simulink model "ASM_FOC_Implementation_Drive2"  (R2021a)
settings: Solver=ode3  StartTime=0.0  StopTime=t_end  FixedStep=dt  RelTol=1e-3  EnableMultiTasking=on
values from neighbouring files (symbols this model uses):
  dt = 5e-6    (= 5e-06)    [Experiment_4_Parameter.m]
  dt_omega = 5e-4    (= 0.0005)    [Experiment_4_Parameter.m]
  EncoderLines = 4096    [Experiment_4_Parameter.m]
  I_N = 4.5*sqrt(2)    [Experiment_4_Parameter.m]
  K_i_i = V_C_i/T_n_i    (= 35.4720958972)    [Experiment_4_Parameter.m]
  K_i_omega = V_C_omega/T_n_omecga_m    (= 32.203207405)    [Experiment_4_Parameter.m]
  K_i_psi = V_C_psi/T_n_psi    (= 3067.48466258)    [Experiment_4_Parameter.m]
  K_p_i = V_C_i    (= 0.195882352941)    [Experiment_4_Parameter.m]
  K_p_omega = V_C_omega    (= 0.32203207405)    [Experiment_4_Parameter.m]
  K_p_psi = V_C_psi    (= 359.636132854)    [Experiment_4_Parameter.m]
  L_m = 0.326    [Experiment_4_Parameter.m]
  L_r = 0.340    (= 0.34)    [Experiment_4_Parameter.m]
  L_s = 0.340    (= 0.34)    [Experiment_4_Parameter.m]
  L_sigma_r = L_r - L_m    (= 0.014)    [Experiment_4_Parameter.m]
  L_sigma_s = L_s - L_m    (= 0.014)    [Experiment_4_Parameter.m]
  M_MN = P_N / omega_N    (= 7.26936072254)    [Experiment_4_Parameter.m]
  n_Igain = 0.075    [Experiment_4_Parameter.m]
  n_Imax = 0.15    [Experiment_4_Parameter.m]
  n_Imin = -n_Imax    (= -0.15)    [Experiment_4_Parameter.m]
  N_N = 2890    [Experiment_4_Parameter.m]
  p = 1    [Experiment_4_Parameter.m]
  Psi_rN = 0.95    [Experiment_4_Parameter.m]
  R_r = 2.9    [Experiment_4_Parameter.m]
  R_s = 2.3    [Experiment_4_Parameter.m]
  sigma = (L_s*L_r - L_m^2)/(L_s*L_r)    (= 0.0806574394464)    [Experiment_4_Parameter.m]
  T_c = 1/4000    (= 0.00025)    [Experiment_4_Parameter.m]
  Theta_M = 0.0022    [Experiment_4_Parameter.m]
  U_dc = 560    [Experiment_4_Parameter.m]
libraries: spsIGBTDiodeLib x6, simulink x3, spsDCVoltageSourceLib x2, spsVoltageMeasurementLib x2, spsGroundLib x1, spspowerguiLib x1, eeTransforms x1
settings Model: Creator=julien  LastModifiedBy=go25bes
settings SolverCC: AlgebraicLoopSolver=TrustRegion
settings DataIOCC: LimitDataPoints=on  SaveFormat=Array  ReturnWorkspaceOutputs=off
settings OptimizationCC: ExpressionDepthLimit=2147483647  LifeSpan=inf
settings DebuggingCC: UnderspecifiedInitializationDetection=Classic  MergeDetectMultiDrivingBlocksExec=none  SolverPrmCheckMsg=warning  MultiTaskRateTransMsg=warning  StateNameClashWarn=warning  SFUnexpectedBacktrackingDiag=warning  SFNoUnconditionalDefaultTransitionDiag=warning  SFExecutionAtInitializationDiag=none  SFMachineParentedDataDiag=warning  ArithmeticOperatorsInVariantConditions=warning
settings HardwareCC: ProdBitPerPointer=32  ProdBitPerSizeT=32  ProdBitPerPtrDiffT=32  ProdLargestAtomicFloat=None  ProdIntDivRoundTo=Undefined  ProdEndianess=Unspecified  ProdWordSize=32  ProdHWDeviceType=32-bit Generic
settings ModelReferenceCC: PropagateSignalLabelsOutOfModel=off
settings SFSimCC: SimUseLocalCustomCode=off  CustomCodeUndefinedFunction=UseInterfaceOnly
settings RTWCC: RTWUseLocalCustomCode=off
settings CodeAppCC: StateflowObjectComments=on
settings GRTTargetCC: TargetLangStandard=C89/C90 (ANSI)
settings ConfigComp: CovMetricSettings=dw  CovSaveCumulativeToWorkspaceVar=on  CovSaveSingleToWorkspaceVar=on  CovExternalEMLEnable=off  CovSFcnEnable=off
settings SimscapeCC: SimscapeNormalizeSystem=off

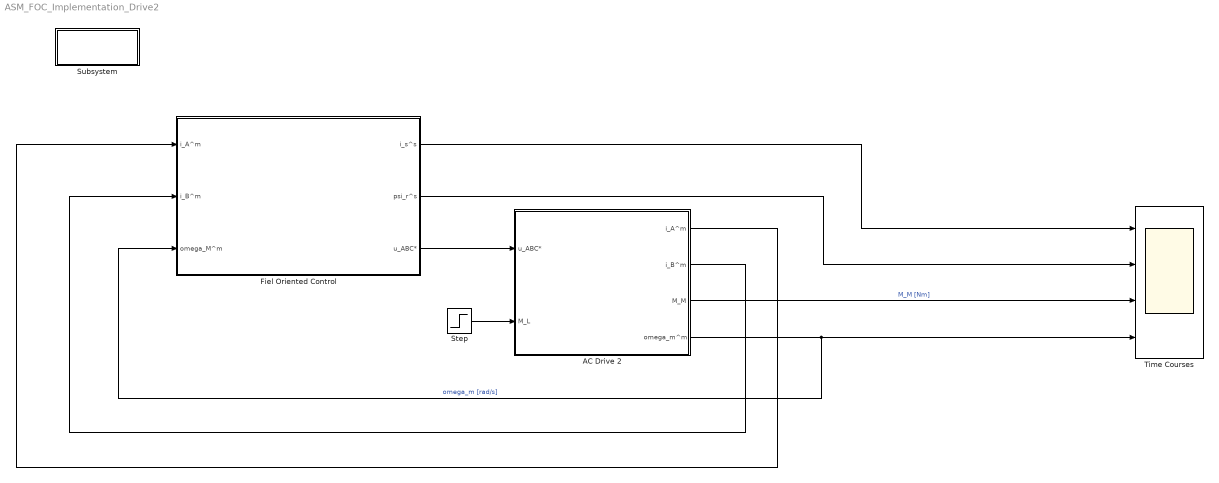
== system ASM_FOC_Implementation_Drive2 ==
  AC Drive 2 : Subsystem
  Fiel Oriented Control : Subsystem
  Step : Step  Time=0.5  After=0.5*M_MN  SampleTime=0
  Subsystem : Subsystem
      settings: OpenFcn=Experiment_4_Parameter
      mask Display: disp('Initialize\n (doppelklicken)')
  Time Courses : Scope  NumInputPorts=4
  wires:
  AC Drive 2/4(omega_m^m) -> Time Courses/4, Fiel Oriented Control/3(omega_M^m)  "omega_m [rad/s]"
  AC Drive 2/3(M_M) -> Time Courses/3  "M_M [Nm]"
  AC Drive 2/1(i_A^m) -> Fiel Oriented Control/1(i_A^m)
  AC Drive 2/2(i_B^m) -> Fiel Oriented Control/2(i_B^m)
  Fiel Oriented Control/1(i_s^s) -> Time Courses/1
  Fiel Oriented Control/3(u_ABC*) -> AC Drive 2/1(u_ABC*)
  Fiel Oriented Control/2(psi_r^s) -> Time Courses/2
  Step/1 -> AC Drive 2/2(M_L)

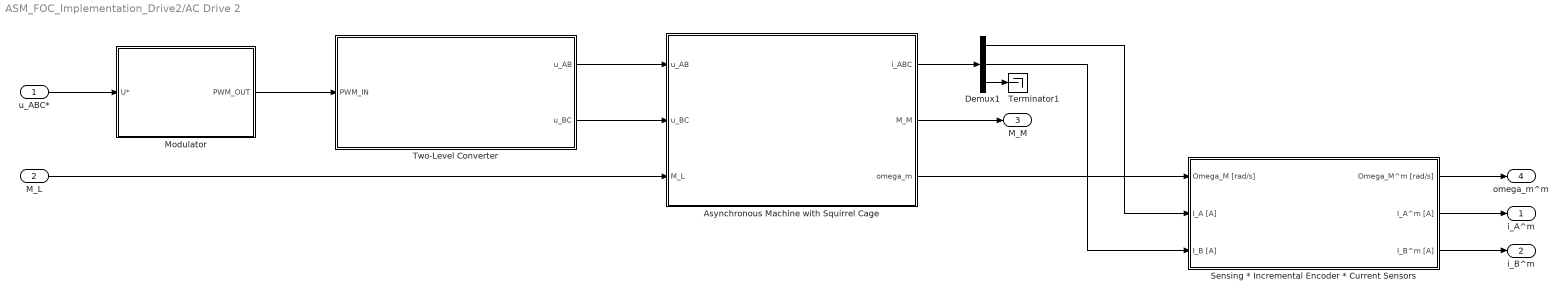
== system ASM_FOC_Implementation_Drive2/AC Drive 2 ==
  u_ABC* : Inport
  M_L : Inport  Port=2
  Asynchronous Machine with Squirrel Cage : Subsystem
  Demux1 : Demux  Outputs=3
  Modulator : Subsystem
  Sensing * Incremental Encoder * Current Sensors : Subsystem
  Terminator1 : Terminator
  Two-Level Converter : Subsystem
  i_A^m : Outport
  i_B^m : Outport  Port=2
  M_M : Outport  Port=3
  omega_m^m : Outport  Port=4
  wires:
  Asynchronous Machine with Squirrel Cage/2(M_M) -> M_M/1
  M_L/1 -> Asynchronous Machine with Squirrel Cage/3(M_L)
  u_ABC*/1 -> Modulator/1(U*)
  Modulator/1(PWM_OUT) -> Two-Level Converter/1(PWM_IN)
  Two-Level Converter/1("u_AB ") -> Asynchronous Machine with Squirrel Cage/1(u_AB)
  Two-Level Converter/2("u_BC ") -> Asynchronous Machine with Squirrel Cage/2(u_BC)
  Asynchronous Machine with Squirrel Cage/1(i_ABC) -> Demux1/1
  Demux1/3 -> Terminator1/1
  Sensing * Incremental Encoder * Current Sensors/1(Omega_M^m [rad/s]) -> omega_m^m/1
  Sensing * Incremental Encoder * Current Sensors/2(I_A^m [A]) -> i_A^m/1
  Demux1/2 -> Sensing * Incremental Encoder * Current Sensors/3(I_B [A])
  Demux1/1 -> Sensing * Incremental Encoder * Current Sensors/2(I_A [A])
  Asynchronous Machine with Squirrel Cage/3(omega_m) -> Sensing * Incremental Encoder * Current Sensors/1(Omega_M [rad/s])
  Sensing * Incremental Encoder * Current Sensors/3(I_B^m [A]) -> i_B^m/1

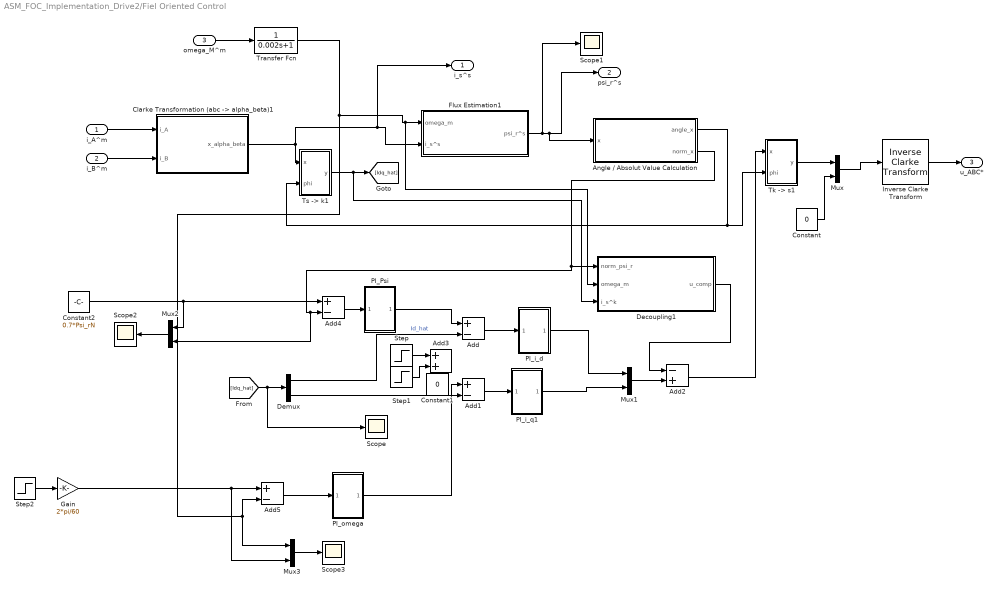
== system ASM_FOC_Implementation_Drive2/Fiel Oriented Control ==
  i_A^m : Inport
  i_B^m : Inport  Port=2
  omega_M^m : Inport  Port=3
  Add{,1,4..5} (4 alike) : Sum  Inputs=+-
  Add2 : Sum  Inputs=-+
  Add3 : Sum
  "Angle / Absolut Value Calculation " : Subsystem
  "Clarke Transformation (abc -> alpha_beta)1" : Subsystem
  Constant : Constant  Value=0
  Constant1 : Constant  Value=0
  Constant2 : Constant  Value=0.7*Psi_rN
  Decoupling1 : Subsystem
  Demux : Demux  Outputs=2
  Flux Estimation1 : Subsystem
  Gain : Gain  Gain=2*pi/60
  Inverse Clarke Transform : eeTransforms/Inverse Clarke Transform  PowerInvariant=off
      settings: SourceProductBaseCode=PS
  Mux{,1..3} (4 alike) : Mux  Inputs=2
  PI_Psi : Subsystem
  PI_i_d : Subsystem
  PI_i_q1 : Subsystem
  PI_omega : Subsystem
  Scope{,1..3} (4 alike) : Scope
  Step : Step  Time=0.6  After=2  SampleTime=0
  Step1 : Step  Time=0.8  After=-2  SampleTime=0
  Step2 : Step  Time=0.2  After=1.1*N_N  SampleTime=0
  "Tk -> s1" : Subsystem
  Transfer Fcn : TransferFcn  Denominator=[0.002 1]
  "Ts -> k1" : Subsystem
  i_s^s : Outport
  psi_r^s : Outport  Port=2
  u_ABC* : Outport  Port=3
  wires:
  i_A^m/1 -> "Clarke Transformation (abc -> alpha_beta)1"/1(i_A)
  i_B^m/1 -> "Clarke Transformation (abc -> alpha_beta)1"/2(i_B)
  "Clarke Transformation (abc -> alpha_beta)1"/1(x_alpha_beta) -> i_s^s/1, Flux Estimation1/2(i_s^s), "Ts -> k1"/1(x)
  Flux Estimation1/1(psi_r^s) -> Scope1/1, "Angle / Absolut Value Calculation "/1(x), psi_r^s/1
  "Tk -> s1"/1(y) -> Mux/1
  "Angle / Absolut Value Calculation "/1(angle_x) -> "Ts -> k1"/2(phi), "Tk -> s1"/2(phi)
  Inverse Clarke Transform/1 -> u_ABC*/1
  Constant/1 -> Mux/2
  Mux/1 -> Inverse Clarke Transform/1
  "Ts -> k1"/1(y) -> Decoupling1/3(i_s^k), [Idq_hat]
  [Idq_hat] -> Scope/1, Demux/1
  Demux/1 -> Add/2  "Id_hat"
  Demux/2 -> Add1/2
  Add/1 -> PI_i_d/1(In1)
  PI_i_d/1(Out1) -> Mux1/1
  Add1/1 -> PI_i_q1/1(In1)
  PI_i_q1/1(Out1) -> Mux1/2
  Mux1/1 -> Add2/2
  Add2/1 -> "Tk -> s1"/1(x)
  "Angle / Absolut Value Calculation "/2(norm_x) -> Mux2/2, Add4/2, Decoupling1/1(norm_psi_r)
  Step/1 -> Add3/1
  Step1/1 -> Add3/2
  Decoupling1/1(u_comp) -> Add2/1
  Add4/1 -> PI_Psi/1(In1)
  Constant2/1 -> Mux2/1, Add4/1
  PI_Psi/1(Out1) -> Add/1
  Mux2/1 -> Scope2/1
  omega_M^m/1 -> Transfer Fcn/1
  Add5/1 -> PI_omega/1(In1)
  PI_omega/1(Out1) -> Add1/1
  Mux3/1 -> Scope3/1
  Step2/1 -> Gain/1
  Gain/1 -> Mux3/2, Add5/1
  Transfer Fcn/1 -> Mux3/1, Add5/2, Decoupling1/2(omega_m), Flux Estimation1/1(omega_m)

== system ASM_FOC_Implementation_Drive2/Subsystem ==

== system ASM_FOC_Implementation_Drive2/AC Drive 2/Asynchronous Machine with Squirrel Cage ==
  u_AB : Inport
  u_BC : Inport  Port=2
  M_L : Inport  Port=3
  Calculation of the Voltage Space Vector : Subsystem
  General AC Machine : Subsystem
  "Inverse Clarke Transformation (alpha_beta -> abc)" : Subsystem
  Rotor Voltage : Constant  Value=0
  Time Courses : Scope  NumInputPorts=5
  i_ABC : Outport
  M_M : Outport  Port=2
  omega_m : Outport  Port=3
  wires:
  Rotor Voltage/1 -> General AC Machine/2(u_r^r)
  Calculation of the Voltage Space Vector/1(u_alpha_beta) -> General AC Machine/1(u_s^s)
  General AC Machine/1(i_s^s) -> Time Courses/1, "Inverse Clarke Transformation (alpha_beta -> abc)"/1(x_alpha_beta)  "i_s^s [A]"
  M_L/1 -> General AC Machine/3(M_L)
  General AC Machine/5(M_M) -> Time Courses/5, M_M/1  "M_M [Nm]"
  "Inverse Clarke Transformation (alpha_beta -> abc)"/1(x_ABC) -> i_ABC/1
  General AC Machine/6(omega_m) -> omega_m/1
  u_AB/1 -> Calculation of the Voltage Space Vector/1(u_AB)
  u_BC/1 -> Calculation of the Voltage Space Vector/2(u_BC)
  General AC Machine/2(psi_s^s) -> Time Courses/2  "psi_s^s [Vs]"
  General AC Machine/3(i_r^r) -> Time Courses/3  "i_r^r [A]"
  General AC Machine/4(psi_r^r) -> Time Courses/4  "psi_r^r [Vs]"

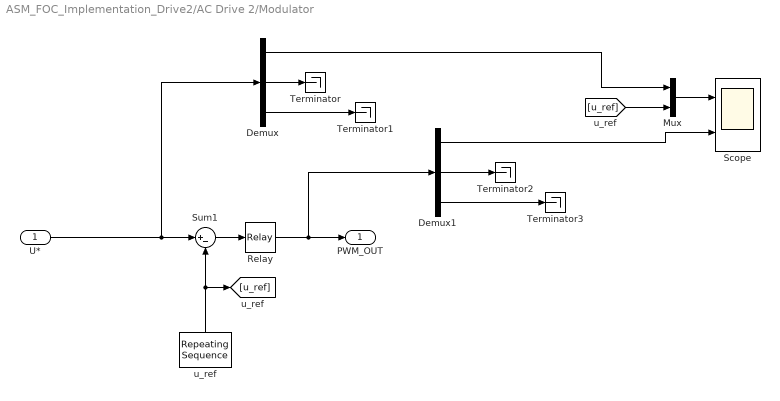
== system ASM_FOC_Implementation_Drive2/AC Drive 2/Modulator ==
  U* : Inport
  Demux : Demux  Outputs=3
  Demux1 : Demux  Outputs=3
  Mux : Mux  Inputs=2
  Relay : Relay  OnSwitchValue=1e-4  OffSwitchValue=-1e-4
  Scope : Scope  NumInputPorts=2
  Sum1 : Sum  Inputs=|+-
  Terminator{,1..3} (4 alike) : Terminator
  u_ref : simulink/Sources/Repeating Sequence  rep_seq_t="[0 T_c/2  T_c]"  rep_seq_y=[1 -1 1]
  PWM_OUT : Outport
  wires:
  Sum1/1 -> Relay/1
  Relay/1 -> Demux1/1, PWM_OUT/1
  Demux/1 -> Mux/1
  Mux/1 -> Scope/1
  u_ref/1 -> [u_ref], Sum1/2
  U*/1 -> Demux/1, Sum1/1
  Demux/2 -> Terminator/1
  Demux/3 -> Terminator1/1
  [u_ref] -> Mux/2
  Demux1/2 -> Terminator2/1
  Demux1/3 -> Terminator3/1
  Demux1/1 -> Scope/2

== system ASM_FOC_Implementation_Drive2/AC Drive 2/Sensing * Incremental Encoder * Current Sensors ==
  Omega_M [rad/s] : Inport
  I_A [A] : Inport  Port=2
  I_B [A] : Inport  Port=3
  Current Sensor : Subsystem  mask(Noise Generator){Noise_Power=0.1*dt, h_Noise=dt, V_Noise=n_Igain, Max_Noise=n_Imax*I_N, Min_Noise=n_Imin*I_N}
      mask prompts: Noise_Power "Noise Power (default: 0.1*h)"; h_Noise "Noise Sampling Time (default: h)"; V_Noise "Noise Gain (Amplification)"; Max_Noise "Maximal Noise Amplitude (Saturation)"; Min_Noise "Minimal Noise Amplitude (Saturation)"
      mask help:
      | This block generates sensor noise (band limited white noise) at a noise sampling time h_Noise [s, default: h] and with a noise power Noise_Power [1, default: 0.1*h], to produce normally distributed bandlimited white noise with a maximal amplitude around 1.
      | The noise amplitude can be amplified with a noise gain V_Noise [1] and saturated with the maximal and minimal noise amplitude selection.
      | With the flag "ENABLE_NOISE" (constant) the noise output can be activated or set to zero.
      mask Display:
      | fprintf('Noise Power: %1.3f [1]\n Noise Sampling Time: %1.3f [s] \n Noise Gain: %g [1] \n Saturation: [%g,%g]'...
      |    ,Noise_Power, h_Noise, V_Noise, Min_Noise, Max_Noise);
      | port_label('input',1,'I [A]');
      | port_label('output',1,'I^m [A]');
  "Current Sensor " : Subsystem  mask(Noise Generator){Noise_Power=0.1*dt, h_Noise=dt, V_Noise=n_Igain, Max_Noise=n_Imax*I_N, Min_Noise=n_Imin*I_N}
      mask prompts: Noise_Power "Noise Power (default: 0.1*h)"; h_Noise "Noise Sampling Time (default: h)"; V_Noise "Noise Gain (Amplification)"; Max_Noise "Maximal Noise Amplitude (Saturation)"; Min_Noise "Minimal Noise Amplitude (Saturation)"
      mask help:
      | This block generates sensor noise (band limited white noise) at a noise sampling time h_Noise [s, default: h] and with a noise power Noise_Power [1, default: 0.1*h], to produce normally distributed bandlimited white noise with a maximal amplitude around 1.
      | The noise amplitude can be amplified with a noise gain V_Noise [1] and saturated with the maximal and minimal noise amplitude selection.
      | With the flag "ENABLE_NOISE" (constant) the noise output can be activated or set to zero.
      mask Display:
      | fprintf('Noise Power: %1.3f [1]\n Noise Sampling Time: %1.3f [s] \n Noise Gain: %g [1] \n Saturation: [%g,%g]'...
      |    ,Noise_Power, h_Noise, V_Noise, Min_Noise, Max_Noise);
      | port_label('input',1,'I [A]');
      | port_label('output',1,'I^m [A]');
  Inkremental-Encoder : Subsystem  mask(Noise Generator){enc_lines=EncoderLines}
      mask prompts: enc_lines "Encoder Lines"
      mask help:
      | This block generates sensor noise (band limited white noise) at a noise sampling time h_Noise [s, default: h] and with a noise power Noise_Power [1, default: 0.1*h], to produce normally distributed bandlimited white noise with a maximal amplitude around 1.
      | The noise amplitude can be amplified with a noise gain V_Noise [1] and saturated with the maximal and minimal noise amplitude selection.
      | With the flag "ENABLE_NOISE" (constant) the noise output can be activated or set to zero.
      mask Display:
      | fprintf('Encoder Lines %g [1]',enc_lines);
      | port_label('input',1,'Omega [rad/s]');
      | port_label('output',1,'Omega^m [rad/s]');
  Omega_M^m [rad/s] : Outport  InitialOutput=0
  I_A^m [A] : Outport  Port=2  InitialOutput=0
  I_B^m [A] : Outport  Port=3  InitialOutput=0
  wires:
  Omega_M [rad/s]/1 -> Inkremental-Encoder/1(Omega [rad/s])
  I_A [A]/1 -> Current Sensor/1(Input)
  I_B [A]/1 -> "Current Sensor "/1(Input)
  "Current Sensor "/1(Output (disturbed by measurement noise)) -> I_B^m [A]/1
  Current Sensor/1(Output (disturbed by measurement noise)) -> I_A^m [A]/1
  Inkremental-Encoder/1(Omega [rad/s] (disturbed by measurement noise)) -> Omega_M^m [rad/s]/1

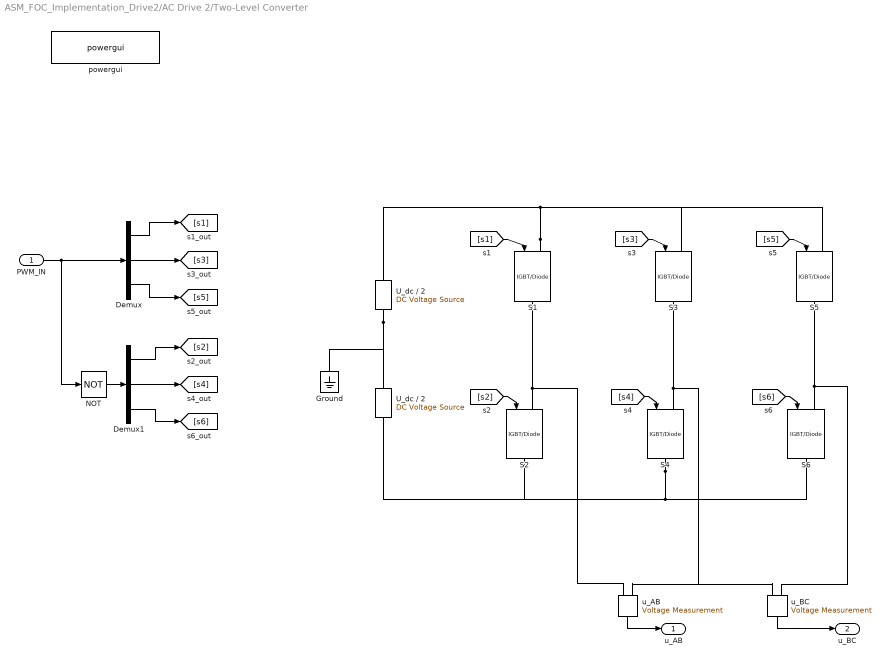
== system ASM_FOC_Implementation_Drive2/AC Drive 2/Two-Level Converter ==
  PWM_IN : Inport
  Demux : Demux  Outputs=3
  Demux1 : Demux  Outputs=3
  Ground : spsGroundLib/Ground  LConnTagsString=a
  NOT : Logic  Operator=NOT  AllPortsSameDT=off  OutDataTypeStr=boolean
  S{1..6} (6 alike) : spsIGBTDiodeLib/IGBT//Diode  Ron=1e-3  Rs=1e5  Cs=inf  Measurements=off
  U_dc / 2 : spsDCVoltageSourceLib/DC Voltage Source  Amplitude=U_dc/2  Measurements=None
  "U_dc / 2 " : spsDCVoltageSourceLib/DC Voltage Source  Amplitude=U_dc/2  Measurements=None
  powergui : spspowerguiLib/powergui  Priority=1  SimulationMode=Discrete  SampleTime=dt  frequency=60  Iterations=50  frequencyindice=0  Pbase=100e6  ErrMax=1e-4  UnitsV=kV  UnitsW=MW  buscounter=0  FunctionMessages=off  echomessages=off  EnableUseOfTLC=off  CurrentSourceSwitches=off  DisableSnubberDevices=off  DisableRonSwitches=off  DisableVfSwitches=off  DisplayEquations=off  AutomaticDiscreteSolvers=off  SolverType=Tustin  Interpol=off  ExternalGateDelay=off  methode=off  Ts=0  x0status=blocks  SPID=off  SwTol=0  HookPort=off  NonlinearTolerance=1e-4  nMaxIteration=100  ContinueOnMaxIteration=off  RestoreLinks=warning  ResistiveCurrentMeasurement=off  Frange=[0:2:500]  Ylog=off  Xlog=on  ShowGrid=off  save=off  variable=ZData  structure=0  ZoomFFT=off  StartTime=0.0  cycles=1  DisplayStyle=1  fundamental=60  FreqAxis=off  MaxFrequency=1000  frequencyindicesteady=1  RmsSteady=1  display=off
  u_AB : spsVoltageMeasurementLib/Voltage Measurement  Tag=PoWeRsYsTeMmEaSuReMeNt  PhasorSimulation=off  OutputType=Magnitude  PSBequivalent=0
  u_BC : spsVoltageMeasurementLib/Voltage Measurement  Tag=PoWeRsYsTeMmEaSuReMeNt  PhasorSimulation=off  OutputType=Magnitude  PSBequivalent=0
  "u_AB " : Outport
  "u_BC " : Outport  Port=2
  wires:
  [s2] -> S2/1
  [s4] -> S4/1
  [s3] -> S3/1
  [s1] -> S1/1
  [s5] -> S5/1
  [s6] -> S6/1
  u_AB/1 -> "u_AB "/1
  u_BC/1 -> "u_BC "/1
  Demux1/2 -> [s4]
  Demux1/3 -> [s6]
  PWM_IN/1 -> NOT/1, Demux/1
  Demux/2 -> [s3]
  Demux1/1 -> [s2]
  NOT/1 -> Demux1/1
  Demux/3 -> [s5]
  Demux/1 -> [s1]
  connections:
  S1/LConn1 -- U_dc / 2/RConn1 -- S5/LConn1 -- S3/LConn1
  S5/RConn1 -- S6/LConn1 -- u_BC/LConn2
  S4/RConn1 -- S6/RConn1 -- S2/RConn1 -- "U_dc / 2 "/LConn1
  U_dc / 2/LConn1 -- Ground/LConn1 -- "U_dc / 2 "/RConn1
  S1/RConn1 -- u_AB/LConn1 -- S2/LConn1
  S3/RConn1 -- u_AB/LConn2 -- u_BC/LConn1 -- S4/LConn1

== system ASM_FOC_Implementation_Drive2/Fiel Oriented Control/Angle // Absolut Value Calculation  ==
  x : Inport
  Demux : Demux  Outputs=2
  Math Function : Math  Operator=square  SignedPower=on  SaturateOnIntegerOverflow=on
  Math Function1 : Math  Operator=square  SignedPower=on  SaturateOnIntegerOverflow=on
  Sqrt : Sqrt  SaturateOnIntegerOverflow=on
  Sum1 : Sum  Inputs=+|+
  Trigonometric Function : Trigonometry  Operator=atan2
  angle_x : Outport
  norm_x : Outport  Port=2
  wires:
  Demux/2 -> Math Function1/1, Trigonometric Function/1
  Demux/1 -> Math Function/1, Trigonometric Function/2
  Trigonometric Function/1 -> angle_x/1
  Math Function1/1 -> Sum1/1
  Sum1/1 -> Sqrt/1
  Math Function/1 -> Sum1/2
  Sqrt/1 -> norm_x/1
  x/1 -> Demux/1

== system ASM_FOC_Implementation_Drive2/Fiel Oriented Control/Clarke Transformation (abc -> alpha_beta)1 ==
  i_A : Inport
  i_B : Inport  Port=2
  2 : Gain  Gain=2
  Mux2 : Mux  Inputs=2
  Sum : Sum  Inputs=++|
  sqrt(3)/3 : Gain  Gain=sqrt(3)/3
  x_alpha_beta : Outport
  wires:
  i_A/1 -> Sum/1, Mux2/1
  i_B/1 -> 2/1
  Sum/1 -> sqrt(3)/3/1
  sqrt(3)/3/1 -> Mux2/2
  Mux2/1 -> x_alpha_beta/1
  2/1 -> Sum/2

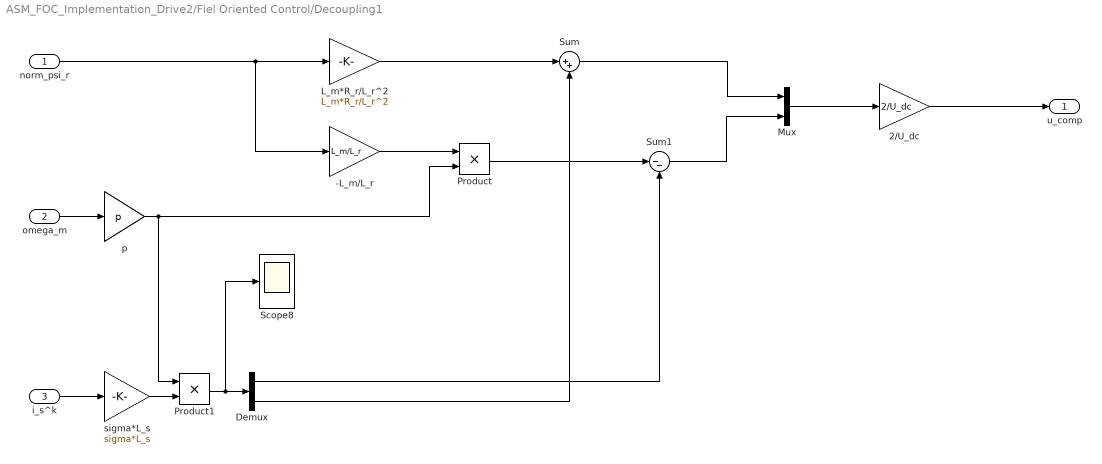
== system ASM_FOC_Implementation_Drive2/Fiel Oriented Control/Decoupling1 ==
  norm_psi_r : Inport
  omega_m : Inport  Port=2
  i_s^k : Inport  Port=3
  -L_m/L_r : Gain  Gain=L_m/L_r
  2/U_dc : Gain  Gain=2/U_dc
  Demux : Demux  Outputs=2
  L_m*R_r/L_r^2 : Gain  Gain=L_m*R_r/L_r^2
  Mux : Mux  Inputs=2
  Product : Product  RndMeth=Zero
  Product1 : Product  RndMeth=Zero
  Scope8 : Scope
  Sum : Sum  Inputs=|++
  Sum1 : Sum  Inputs=|--
  p : Gain  Gain=p
  sigma*L_s : Gain  Gain=sigma*L_s
  u_comp : Outport
  wires:
  omega_m/1 -> p/1
  norm_psi_r/1 -> -L_m/L_r/1, L_m*R_r/L_r^2/1
  i_s^k/1 -> sigma*L_s/1
  -L_m/L_r/1 -> Product/1
  p/1 -> Product1/1, Product/2
  sigma*L_s/1 -> Product1/2
  Product1/1 -> Scope8/1, Demux/1
  L_m*R_r/L_r^2/1 -> Sum/1
  Demux/2 -> Sum/2
  Product/1 -> Sum1/1
  Demux/1 -> Sum1/2
  Mux/1 -> 2/U_dc/1
  Sum/1 -> Mux/1
  Sum1/1 -> Mux/2
  2/U_dc/1 -> u_comp/1

== system ASM_FOC_Implementation_Drive2/Fiel Oriented Control/Flux Estimation1 ==
  omega_m : Inport
  i_s^s : Inport  Port=2
  Integrator : Integrator
  J : Subsystem
  L_m : Gain  Gain=L_m
  Product : Product  RndMeth=Zero
  R_r/L_r : Gain  Gain=R_r/L_r
  Sum : Sum  Inputs=++|
  Sum1 : Sum  Inputs=|+-
  p : Gain  Gain=p
  psi_r^s : Outport
  wires:
  L_m/1 -> Sum1/1
  Product/1 -> J/1(x)
  J/1(Jx) -> Sum/1
  i_s^s/1 -> L_m/1
  Sum/1 -> Integrator/1
  R_r/L_r/1 -> Sum/2
  Sum1/1 -> R_r/L_r/1
  Integrator/1 -> psi_r^s/1, Sum1/2, Product/2
  omega_m/1 -> p/1
  p/1 -> Product/1

== system ASM_FOC_Implementation_Drive2/Fiel Oriented Control/PI_Psi ==
  In1 : Inport
  Add : Sum  Inputs=+-
  Add1 : Sum  Inputs=+-
  Add2 : Sum
  Gain : Gain  Gain=K_p_psi
  Gain1add : Gain  Gain=K_i_psi
  Gain2 : Gain  Gain=7
  Integrator : Integrator
  Saturation : Saturate  UpperLimit=1.5*I_N  LowerLimit=-1.5*I_N
  Out1 : Outport
  wires:
  In1/1 -> Gain1add/1, Gain/1
  Gain/1 -> Add2/1
  Integrator/1 -> Add2/2
  Add2/1 -> Saturation/1, Add/1
  Saturation/1 -> Add/2, Out1/1
  Add/1 -> Gain2/1
  Gain2/1 -> Add1/2
  Gain1add/1 -> Add1/1
  Add1/1 -> Integrator/1

== system ASM_FOC_Implementation_Drive2/Fiel Oriented Control/PI_i_d ==
  In1 : Inport
  Add2 : Sum
  Gain : Gain  Gain=K_p_i
  Gain1 : Gain  Gain=K_i_i
  Integrator : Integrator
  Out1 : Outport
  wires:
  In1/1 -> Gain1/1, Gain/1
  Gain1/1 -> Integrator/1
  Gain/1 -> Add2/1
  Integrator/1 -> Add2/2
  Add2/1 -> Out1/1

== system ASM_FOC_Implementation_Drive2/Fiel Oriented Control/PI_i_q1 ==
  In1 : Inport
  Add2 : Sum
  Gain : Gain  Gain=K_p_i
  Gain1 : Gain  Gain=K_i_i
  Integrator : Integrator
  Out1 : Outport
  wires:
  In1/1 -> Gain1/1, Gain/1
  Gain1/1 -> Integrator/1
  Gain/1 -> Add2/1
  Integrator/1 -> Add2/2
  Add2/1 -> Out1/1

== system ASM_FOC_Implementation_Drive2/Fiel Oriented Control/PI_omega ==
  In1 : Inport
  Add : Sum  Inputs=+-
  Add1 : Sum  Inputs=+-
  Add2 : Sum
  Gain : Gain  Gain=K_p_omega
  Gain1add : Gain  Gain=K_i_omega
  Gain2 : Gain  Gain=20000
  Integrator : Integrator
  Saturation : Saturate  UpperLimit=1.5*I_N  LowerLimit=-1.5*I_N
  Out1 : Outport
  wires:
  In1/1 -> Gain1add/1, Gain/1
  Gain/1 -> Add2/1
  Integrator/1 -> Add2/2
  Add2/1 -> Saturation/1, Add/1
  Saturation/1 -> Add/2, Out1/1
  Add/1 -> Gain2/1
  Gain2/1 -> Add1/2
  Gain1add/1 -> Add1/1
  Add1/1 -> Integrator/1

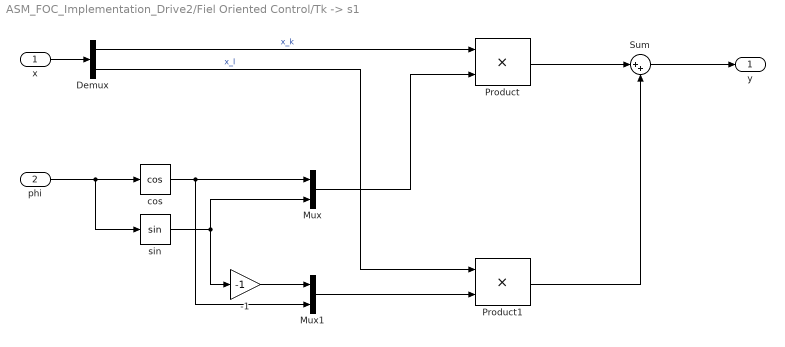
== system ASM_FOC_Implementation_Drive2/Fiel Oriented Control/Tk -> s1 ==
  x : Inport
  phi : Inport  Port=2
  -1 : Gain  Gain=-1
  Demux : Demux  Outputs=2
  Mux : Mux  Inputs=2
  Mux1 : Mux  Inputs=2
  Product : Product  RndMeth=Zero
  Product1 : Product  RndMeth=Zero
  Sum : Sum  Inputs=|++
  cos : Trigonometry  Operator=cos
  sin : Trigonometry
  y : Outport
  wires:
  x/1 -> Demux/1
  phi/1 -> cos/1, sin/1
  cos/1 -> Mux/1, Mux1/2
  sin/1 -> Mux/2, -1/1
  Mux/1 -> Product/2
  -1/1 -> Mux1/1
  Mux1/1 -> Product1/2
  Demux/2 -> Product1/1  "x_l"
  Product/1 -> Sum/1
  Product1/1 -> Sum/2
  Sum/1 -> y/1
  Demux/1 -> Product/1  "x_k"

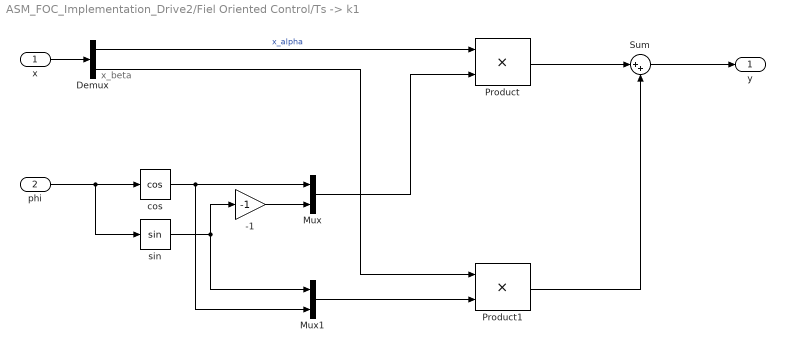
== system ASM_FOC_Implementation_Drive2/Fiel Oriented Control/Ts -> k1 ==
  note: x_beta
  x : Inport
  phi : Inport  Port=2
  -1 : Gain  Gain=-1
  Demux : Demux  Outputs=2
  Mux : Mux  Inputs=2
  Mux1 : Mux  Inputs=2
  Product : Product  RndMeth=Zero
  Product1 : Product  RndMeth=Zero
  Sum : Sum  Inputs=|++
  cos : Trigonometry  Operator=cos
  sin : Trigonometry
  y : Outport
  wires:
  x/1 -> Demux/1
  phi/1 -> cos/1, sin/1
  Demux/1 -> Product/1  "x_alpha"
  cos/1 -> Mux/1, Mux1/2
  sin/1 -> -1/1, Mux1/1
  Mux/1 -> Product/2
  Mux1/1 -> Product1/2
  Demux/2 -> Product1/1
  Product/1 -> Sum/1
  Product1/1 -> Sum/2
  -1/1 -> Mux/2
  Sum/1 -> y/1

== system ASM_FOC_Implementation_Drive2/AC Drive 2/Asynchronous Machine with Squirrel Cage/Calculation of the Voltage Space Vector ==
  u_AB : Inport
  u_BC : Inport  Port=2
  1/3 : Gain  Gain=1/3
  2/3 : Gain  Gain=2/3
  Mux2 : Mux  Inputs=2
  Sum : Sum  Inputs=|++
  sqrt(3)/3 : Gain  Gain=sqrt(3)/3
  u_alpha_beta : Outport
  wires:
  Mux2/1 -> u_alpha_beta/1
  u_AB/1 -> 2/3/1
  u_BC/1 -> sqrt(3)/3/1, 1/3/1
  2/3/1 -> Sum/1
  1/3/1 -> Sum/2
  Sum/1 -> Mux2/1
  sqrt(3)/3/1 -> Mux2/2

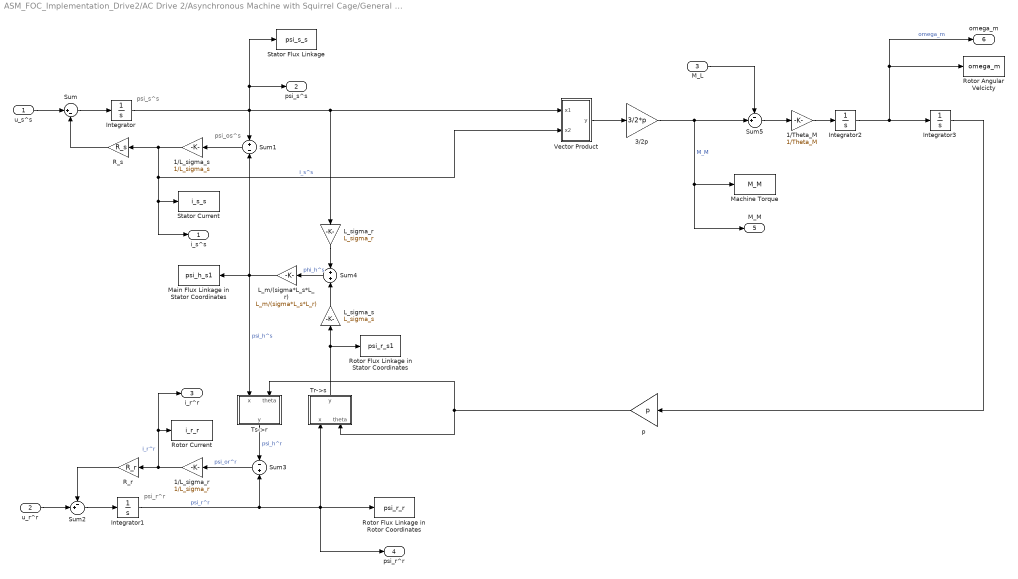
== system ASM_FOC_Implementation_Drive2/AC Drive 2/Asynchronous Machine with Squirrel Cage/General AC Machine ==
  note: psi_s^s
  note: psi_r^r
  note: psi_os^s
  u_s^s : Inport
  u_r^r : Inport  Port=2
  M_L : Inport  Port=3
  1/L_sigma_r : Gain  Gain=1/L_sigma_r
  1/L_sigma_s : Gain  Gain=1/L_sigma_s
  1/Theta_M : Gain  Gain=1/Theta_M
  3/2p : Gain  Gain=3/2*p
  Integrator{,1..3} (4 alike) : Integrator
  L_m/(sigma*L_s*L_r) : Gain  Gain=L_m/(sigma*L_s*L_r)
  L_sigma_r : Gain  Gain=L_sigma_r
  L_sigma_s : Gain  Gain=L_sigma_s
  Machine Torque : ToWorkspace  VariableName=M_M  SaveFormat=Timeseries  SampleTime=-1
  "Main Flux Linkage in Stator Coordinates " : ToWorkspace  VariableName=psi_h_s1  SaveFormat=Timeseries  SampleTime=-1
  R_r : Gain  Gain=R_r
  R_s : Gain  Gain=R_s
  Rotor Angular Velcicty : ToWorkspace  VariableName=omega_m  SaveFormat=Timeseries  SampleTime=-1
  Rotor Current : ToWorkspace  VariableName=i_r_r  SaveFormat=Timeseries  SampleTime=-1
  Rotor Flux Linkage in Rotor Coordinates : ToWorkspace  VariableName=psi_r_r  SaveFormat=Timeseries  SampleTime=-1
  "Rotor Flux Linkage in Stator Coordinates " : ToWorkspace  VariableName=psi_r_s1  SaveFormat=Timeseries  SampleTime=-1
  Stator Current : ToWorkspace  VariableName=i_s_s  SaveFormat=Timeseries  SampleTime=-1
  Stator Flux Linkage : ToWorkspace  VariableName=psi_s_s  SaveFormat=Timeseries  SampleTime=-1
  Sum : Sum  Inputs=|+-
  Sum1 : Sum  Inputs=+|-
  Sum2 : Sum  Inputs=-+|
  Sum3 : Sum  Inputs=-|+
  Sum4 : Sum  Inputs=+|+
  Sum5 : Sum  Inputs=-+|
  Tr->s : Subsystem
  Ts->r : Subsystem
  Vector Product : Subsystem
  p : Gain  Gain=p
  i_s^s : Outport
  psi_s^s : Outport  Port=2
  i_r^r : Outport  Port=3
  psi_r^r : Outport  Port=4
  M_M : Outport  Port=5
  omega_m : Outport  Port=6
  wires:
  u_s^s/1 -> Sum/1
  R_s/1 -> Sum/2
  Sum/1 -> Integrator/1
  1/L_sigma_s/1 -> R_s/1, Stator Current/1, i_s^s/1, Vector Product/2(x2)  "i_s^s"
  Integrator/1 -> psi_s^s/1, Stator Flux Linkage/1, Sum1/1, L_sigma_r/1, Vector Product/1(x1)
  Sum1/1 -> 1/L_sigma_s/1
  u_r^r/1 -> Sum2/2
  Sum2/1 -> Integrator1/1
  R_r/1 -> Sum2/1
  1/L_sigma_r/1 -> R_r/1, Rotor Current/1, i_r^r/1  "i_r^r"
  Integrator1/1 -> Sum3/2, psi_r^r/1, Tr->s/1(x), Rotor Flux Linkage in Rotor Coordinates/1  "psi_r^r"
  Sum3/1 -> 1/L_sigma_r/1  "psi_or^r"
  Tr->s/1(y) -> "Rotor Flux Linkage in Stator Coordinates "/1, L_sigma_s/1
  L_sigma_r/1 -> Sum4/1
  L_sigma_s/1 -> Sum4/2
  Vector Product/1(y) -> 3/2p/1
  3/2p/1 -> Machine Torque/1, M_M/1, Sum5/2  "M_M"
  M_L/1 -> Sum5/1
  Sum5/1 -> 1/Theta_M/1
  1/Theta_M/1 -> Integrator2/1
  Integrator2/1 -> Integrator3/1, Rotor Angular Velcicty/1, omega_m/1  "omega_m"
  Integrator3/1 -> p/1
  Ts->r/1(y) -> Sum3/1  "psi_h^r"
  L_m/(sigma*L_s*L_r)/1 -> "Main Flux Linkage in Stator Coordinates "/1, Sum1/2, Ts->r/1(x)  "psi_h^s"
  p/1 -> Ts->r/2(theta), Tr->s/2(theta)
  Sum4/1 -> L_m/(sigma*L_s*L_r)/1  "phi_h^s"

== system ASM_FOC_Implementation_Drive2/AC Drive 2/Asynchronous Machine with Squirrel Cage/Inverse Clarke Transformation (alpha_beta -> abc) ==
  x_alpha_beta : Inport
  "1/2 " : Gain  Gain=1/2
  Demux : Demux  Outputs=2
  Mux2 : Mux  Inputs=3
  Sum : Sum  Inputs=|-+
  Sum1 : Sum  Inputs=|--
  sqrt(3)/2 : Gain  Gain=sqrt(3)/2
  x_ABC : Outport
  wires:
  x_alpha_beta/1 -> Demux/1
  Demux/1 -> Mux2/1, "1/2 "/1
  Mux2/1 -> x_ABC/1
  Demux/2 -> sqrt(3)/2/1
  "1/2 "/1 -> Sum/1, Sum1/1
  sqrt(3)/2/1 -> Sum/2, Sum1/2
  Sum/1 -> Mux2/2
  Sum1/1 -> Mux2/3

== system ASM_FOC_Implementation_Drive2/AC Drive 2/Sensing * Incremental Encoder * Current Sensors/Current Sensor ==
  Input : Inport
  Add : Sum
  Band-Limited White Noise : simulink/Sources/Band-Limited White Noise  Cov=[Noise_Power]  Ts=h_Noise  seed=[23341]
  Gain26 : Gain  Gain=V_Noise
  Rate Transition : RateTransition  OutPortSampleTime=h_Noise
  Saturation : Saturate  UpperLimit=Max_Noise  LowerLimit=Min_Noise
  Output (disturbed by measurement noise) : Outport
  wires:
  Saturation/1 -> Add/2
  Input/1 -> Add/1
  Rate Transition/1 -> Gain26/1
  Gain26/1 -> Saturation/1
  Band-Limited White Noise/1 -> Rate Transition/1
  Add/1 -> Output (disturbed by measurement noise)/1

== system ASM_FOC_Implementation_Drive2/AC Drive 2/Sensing * Incremental Encoder * Current Sensors/Current Sensor  ==
  Input : Inport
  Add : Sum
  Band-Limited White Noise : simulink/Sources/Band-Limited White Noise  Cov=[Noise_Power]  Ts=h_Noise  seed=[23341]
  Gain26 : Gain  Gain=V_Noise
  Rate Transition : RateTransition  OutPortSampleTime=h_Noise
  Saturation : Saturate  UpperLimit=Max_Noise  LowerLimit=Min_Noise
  Output (disturbed by measurement noise) : Outport
  wires:
  Band-Limited White Noise/1 -> Rate Transition/1
  Gain26/1 -> Saturation/1
  Rate Transition/1 -> Gain26/1
  Input/1 -> Add/1
  Saturation/1 -> Add/2
  Add/1 -> Output (disturbed by measurement noise)/1

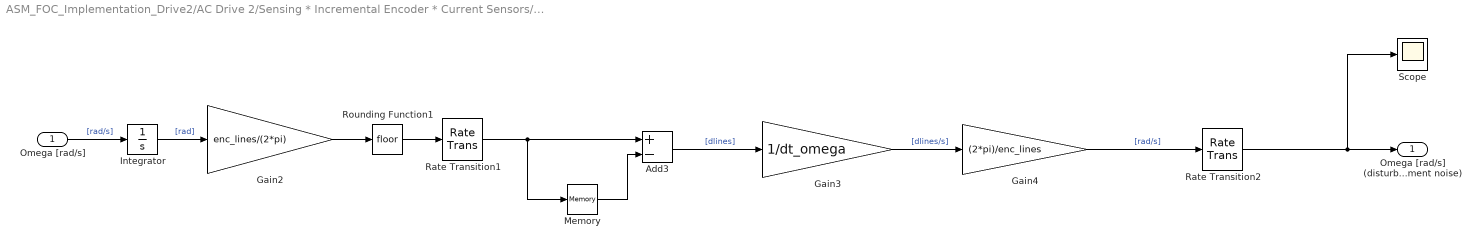
== system ASM_FOC_Implementation_Drive2/AC Drive 2/Sensing * Incremental Encoder * Current Sensors/Inkremental-Encoder ==
  Omega [rad/s] : Inport
  Add3 : Sum  Inputs=+-
  Gain2 : Gain  Gain=enc_lines/(2*pi)
  Gain3 : Gain  Gain=1/dt_omega
  Gain4 : Gain  Gain=(2*pi)/enc_lines
  Integrator : Integrator
  Memory : Memory  InheritSampleTime=on
  Rate Transition1 : RateTransition  OutPortSampleTime=dt_omega
  Rate Transition2 : RateTransition  OutPortSampleTime=dt
  Rounding Function1 : Rounding
  Scope : Scope
  Omega [rad/s] (disturbed by measurement noise) : Outport
  wires:
  Integrator/1 -> Gain2/1  "[rad]"
  Gain2/1 -> Rounding Function1/1
  Memory/1 -> Add3/2
  Add3/1 -> Gain3/1  "[dlines]"
  Gain3/1 -> Gain4/1  "[dlines/s]"
  Gain4/1 -> Rate Transition2/1  "[rad/s]"
  Rounding Function1/1 -> Rate Transition1/1
  Omega [rad/s]/1 -> Integrator/1  "[rad/s]"
  Rate Transition1/1 -> Memory/1, Add3/1
  Rate Transition2/1 -> Omega [rad/s] (disturbed by measurement noise)/1, Scope/1

== system ASM_FOC_Implementation_Drive2/Fiel Oriented Control/Flux Estimation1/J ==
  note: x_beta
  x : Inport
  -1 : Gain  Gain=-1
  Demux : Demux  Outputs=2
  Mux : Mux  Inputs=2
  Jx : Outport
  wires:
  x/1 -> Demux/1
  Demux/1 -> Mux/2  "x_alpha"
  Demux/2 -> -1/1
  Mux/1 -> Jx/1
  -1/1 -> Mux/1

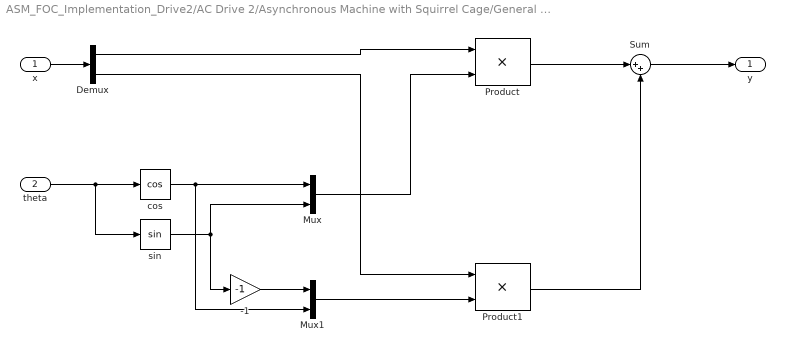
== system ASM_FOC_Implementation_Drive2/AC Drive 2/Asynchronous Machine with Squirrel Cage/General AC Machine/Tr->s ==
  x : Inport
  theta : Inport  Port=2
  -1 : Gain  Gain=-1
  Demux : Demux  Outputs=2
  Mux : Mux  Inputs=2
  Mux1 : Mux  Inputs=2
  Product : Product  RndMeth=Zero
  Product1 : Product  RndMeth=Zero
  Sum : Sum  Inputs=|++
  cos : Trigonometry  Operator=cos
  sin : Trigonometry
  y : Outport
  wires:
  x/1 -> Demux/1
  theta/1 -> cos/1, sin/1
  cos/1 -> Mux/1, Mux1/2
  sin/1 -> Mux/2, -1/1
  Mux/1 -> Product/2
  -1/1 -> Mux1/1
  Mux1/1 -> Product1/2
  Demux/2 -> Product1/1
  Product/1 -> Sum/1
  Product1/1 -> Sum/2
  Sum/1 -> y/1
  Demux/1 -> Product/1

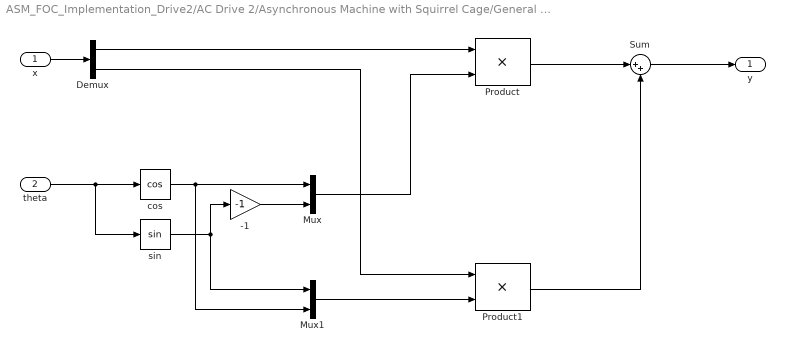
== system ASM_FOC_Implementation_Drive2/AC Drive 2/Asynchronous Machine with Squirrel Cage/General AC Machine/Ts->r ==
  x : Inport
  theta : Inport  Port=2
  -1 : Gain  Gain=-1
  Demux : Demux  Outputs=2
  Mux : Mux  Inputs=2
  Mux1 : Mux  Inputs=2
  Product : Product  RndMeth=Zero
  Product1 : Product  RndMeth=Zero
  Sum : Sum  Inputs=|++
  cos : Trigonometry  Operator=cos
  sin : Trigonometry
  y : Outport
  wires:
  x/1 -> Demux/1
  theta/1 -> cos/1, sin/1
  Demux/1 -> Product/1
  cos/1 -> Mux/1, Mux1/2
  sin/1 -> -1/1, Mux1/1
  Mux/1 -> Product/2
  Mux1/1 -> Product1/2
  Demux/2 -> Product1/1
  Product/1 -> Sum/1
  Product1/1 -> Sum/2
  -1/1 -> Mux/2
  Sum/1 -> y/1

== system ASM_FOC_Implementation_Drive2/AC Drive 2/Asynchronous Machine with Squirrel Cage/General AC Machine/Vector Product ==
  x1 : Inport
  x2 : Inport  Port=2
  Demux : Demux  Outputs=2
  Demux1 : Demux  Outputs=2
  Product : Product  RndMeth=Zero
  Product1 : Product  RndMeth=Zero
  Sum : Sum  Inputs=|+-
  y : Outport
  wires:
  Sum/1 -> y/1
  Product1/1 -> Sum/2
  Product/1 -> Sum/1
  Demux1/1 -> Product1/2
  Demux/2 -> Product1/1
  Demux1/2 -> Product/2
  Demux/1 -> Product/1
  x2/1 -> Demux1/1
  x1/1 -> Demux/1
